simulink model "phiupdate_new"  (R2018b)
settings: Solver=VariableStepAuto  StartTime=0.0  StopTime=10.0  RelTol=1e-3
undefined symbols (not defined in the file or in its folder): g, phi, s, Torque
settings Model: Creator=mishray  LastModifiedBy=mishray

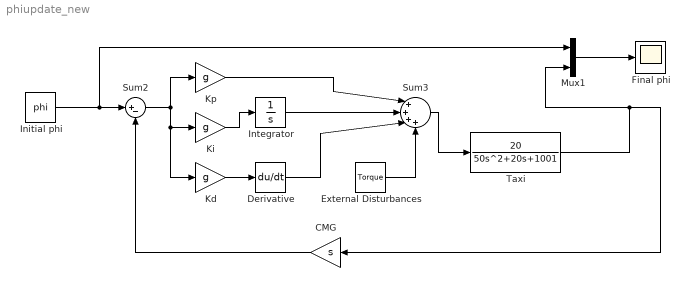
== system phiupdate_new ==
  CMG : Gain  Gain=s
  Derivative : Derivative
  External Disturbances : Constant  Value=Torque
  Final phi : Scope
  Initial phi : Constant  Value=phi
  Integrator : Integrator
  "Kd " : Gain  Gain=g
  "Ki " : Gain  Gain=g
  Kp : Gain  Gain=g
  Mux1 : Mux  Inputs=2
  Sum2 : Sum  Inputs=|+-
  Sum3 : Sum  Inputs=|++++
  Taxi : TransferFcn  Numerator=[20]  Denominator=[50 20 1001]
  wires:
  Taxi/1 -> Mux1/2, CMG/1
  Sum3/1 -> Taxi/1
  CMG/1 -> Sum2/2
  Sum2/1 -> "Kd "/1, "Ki "/1, Kp/1
  Kp/1 -> Sum3/1
  Initial phi/1 -> Mux1/1, Sum2/1
  External Disturbances/1 -> Sum3/4
  Mux1/1 -> Final phi/1
  "Ki "/1 -> Integrator/1
  Integrator/1 -> Sum3/2
  "Kd "/1 -> Derivative/1
  Derivative/1 -> Sum3/3
